simulink model "power_10MW5_diode"  (R2023b)
settings: Solver=FixedStepDiscrete  StartTime=0.0  StopTime=2.6  RelTol=1e-3
InitFcn:
  | power_sysinit
StopFcn:
  | ans = [pl_T1(end),max(tem_T1),pl_T2(end),max(tem_T2),pl_D1(end),max(tem_D1),...
  |     pl_D2(end),max(tem_D2),pl_D5(end),max(tem_D5),i_45(end),i_15(end),pl_D7(end),max(tem_D7)]
values from neighbouring files (symbols this model uses):
  C_absorption = 34e-6    (= 3.4e-05)    [power_sysinit.m]
  f = 40    [power_sysinit.m]
  f_switch = 900    [power_sysinit.m]
  IN = 0.3    [power_sysinit.m]
  L_absorption = 4e-6    (= 4e-06)    [power_sysinit.m]
  m = 1/75*f    (= 0.533333333333)    [power_sysinit.m]
  PM = 0    [power_sysinit.m]
  R_absorption = 0.45    [power_sysinit.m]
  TC = 1/f_switch    (= 0.00111111111111)    [power_sysinit.m]
  temp_init = 40    [power_sysinit.m]
  Ts1 = 1e-6    (= 1e-06)    [power_sysinit.m]
  Ts2 = 500E-6    (= 0.0005)    [power_sysinit.m]
  Udc = 2500    [power_sysinit.m]
undefined symbols (not defined in the file or in its folder): DIODE_204520, DIODE_344520, DIODE_364520, DIODE_364521, DIODE_D1031SH, DIODE_D1331SH, IGCT_364520_36, IGCT_364521_36, IGCT_654522_6, magnitude, Rth_h, Rth_h_tau
libraries: spsMeanLib x138, simulink x32, spsSeriesRLCBranchLib x30, spsRMSLib x24, spsCurrentMeasurementLib x21, dspstat3 x13, spsDiodeLib x12, spsVoltageMeasurementLib x12, spsOnDelayLib x6, powerlib_extras x5, spsDCVoltageSourceLib x4, spsIGBTDiodeLib x4
(part 1 of 6)
settings Model: SimulationMode=accelerator  Creator=tk  LastModifiedBy=Jhchen
settings SolverCC: AlgebraicLoopSolver=TrustRegion
settings DataIOCC: ReturnWorkspaceOutputs=off
settings OptimizationCC: EfficientMapNaN2IntZero=off
settings DebuggingCC: UnconnectedInputMsg=warning  UnconnectedOutputMsg=warning  UnconnectedLineMsg=warning  ArithmeticOperatorsInVariantConditions=warning
settings HardwareCC: TargetBitPerPointer=64  TargetBitPerSizeT=64  TargetBitPerPtrDiffT=64  TargetLongLongMode=on  TargetIntDivRoundTo=Zero  TargetEndianess=LittleEndian  TargetWordSize=64  TargetHWDeviceType=MATLAB Host  ProdEqTarget=off
settings ModelReferenceCC: EnableRefExpFcnMdlSchedulingChecks=on
settings SFSimCC: CustomCodeUndefinedFunction=UseInterfaceOnly
settings RTWCC: DLArmComputeVersion=19.05
settings CodeAppCC: MaxIdLength=128
settings GRTTargetCC: TargetLangStandard=C89/C90 (ANSI)  CombineOutputUpdateFcns=off  GRTInterface=on

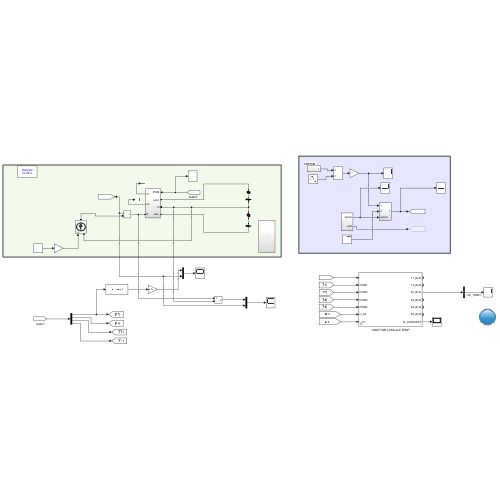
[thumbnail: Simulink's stored preview of the top-level diagram]
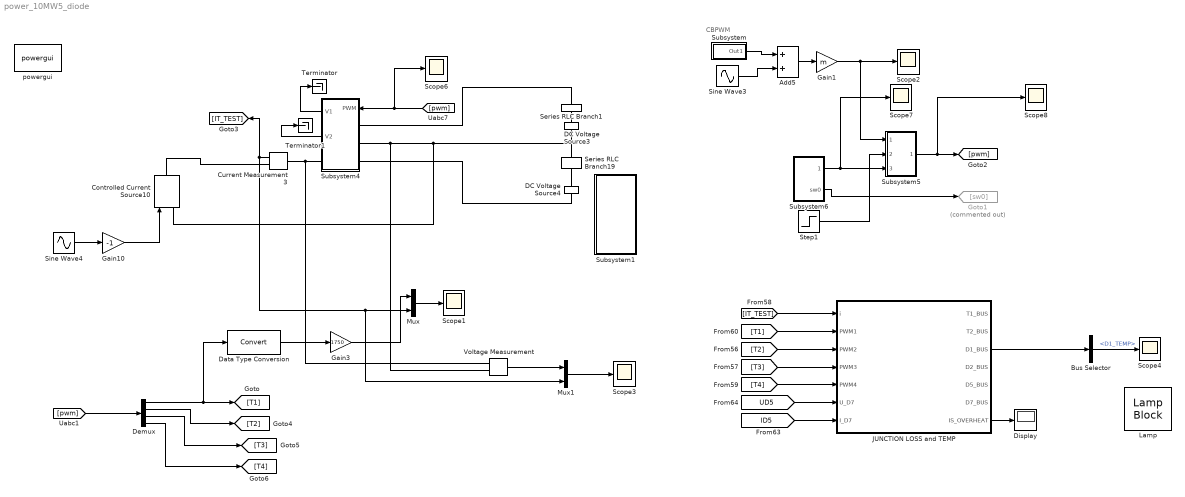
== system power_10MW5_diode ==
  note: CBPWM
  Add5 : Sum
  Bus Selector : BusSelector  OutputSignals=D1_TEMP
  Controlled Current Source10 : spsControlledCurrentSourceLib/Controlled Current Source  Initialize=on  Source_Type=DC  Amplitude=0  Phase=0  Frequency=0  Measurements=None
  Current Measurement3 : spsCurrentMeasurementLib/Current Measurement  PhasorSimulation=off  OutputType=Complex  PSBequivalent=0
  DC Voltage Source3 : spsDCVoltageSourceLib/DC Voltage Source  Amplitude=2500  Measurements=None
  DC Voltage Source4 : spsDCVoltageSourceLib/DC Voltage Source  Amplitude=2500  Measurements=None
  Data Type Conversion : DataTypeConversion  SaturateOnIntegerOverflow=off  RndMeth=Floor
  Demux : Demux
  Display : Display
  Gain1 : Gain  Gain=m
  Gain10 : Gain  Gain=-1
  Gain3 : Gain  Gain=1750
  Goto1 : Goto  Commented=on  GotoTag=sw0
  JUNCTION LOSS and TEMP : Subsystem  mask{DIODE_TYPE=34L4520, IGCT_TYPE=65l4522}
      mask prompts: DIODE_TYPE "DIODE"; IGCT_TYPE "IGCT"
      mask TypeOptions IGCT_TYPE: 65l4522 | 36L4520 | 36L4521
      mask DialogControl DescGroupVar Prompt: JUNCTION LOSS and TEMP
      mask DialogControl DescTextVar Prompt: 功率器件损耗与结温估算模块。通过下拉菜单选择相应IGCT与二极管
      mask DialogControl ParameterGroupVar Prompt: 参数
      mask DialogControl Container4 Prompt: IGCT型号，其中36L4520与36L4521为二极管和IGCT共用
  Lamp : LampBlock  LabelPosition=Hide
  Mux : Mux  Inputs=2
  Mux1 : Mux  Inputs=2
  Scope{1..4,6..8} (7 alike) : Scope
  Series RLC Branch1 : spsSeriesRLCBranchLib/Series RLC Branch  LConnTagsString=__new0  RConnTagsString=__new0  BranchType=R  Resistance=1E-6  Inductance=1e-3  SetiL0=off  InitialCurrent=0  Capacitance=1e-6  Setx0=off  InitialVoltage=0  Measurements=None
  Series RLC Branch19 : spsSeriesRLCBranchLib/Series RLC Branch  LConnTagsString=__new0  RConnTagsString=__new0  BranchType=R  Resistance=1E-6  Inductance=1e-3  SetiL0=off  InitialCurrent=0  Capacitance=1e-6  Setx0=off  InitialVoltage=0  Measurements=None
  Sine Wave3 : Sin  Frequency=2*f*pi  SampleTime=Ts2
  Sine Wave4 : Sin  Amplitude=IN*1750*1.4142  Frequency=2*f*pi  Phase=pi*(-0.05*f/50)  SampleTime=Ts1
  Step1 : Step  Time=0.00001  SampleTime=0
  Subsystem : Subsystem
  Subsystem1 : Subsystem
  Subsystem4 : Subsystem
  Subsystem5 : Subsystem
  Subsystem6 : Subsystem
  Terminator : Terminator
  Terminator1 : Terminator
  Voltage Measurement : spsVoltageMeasurementLib/Voltage Measurement  PhasorSimulation=off  OutputType=Complex  PSBequivalent=0
  powergui : sps_lib/powergui  Priority=1  SimulationMode=Discrete  SampleTime=1e-6  frequency=60  Iterations=50  frequencyindice=0  Pbase=100e6  ErrMax=1e-4  UnitsV=kV  UnitsW=MW  buscounter=0  FunctionMessages=off  echomessages=off  EnableUseOfTLC=off  CurrentSourceSwitches=off  DisableSnubberDevices=off  DisableRonSwitches=off  DisableVfSwitches=off  DisplayEquations=off  AutomaticDiscreteSolvers=off  SolverType=Tustin/Backward Euler (TBE)  Interpol=off  ExternalGateDelay=off  methode=off  Ts=100  x0status=blocks  SPID=off  SwTol=0  HookPort=off  NonlinearTolerance=1e-4  nMaxIteration=100  ContinueOnMaxIteration=off  RestoreLinks=warning  ResistiveCurrentMeasurement=off  Frange=[0:2:500]  Ylog=off  Xlog=on  ShowGrid=off  save=off  variable=ZData  structure=Iabc  ZoomFFT=off  StartTime=5.3  cycles=1  DisplayStyle=2  fundamental=47.875  FreqAxis=off  MaxFrequency=2000  frequencyindicesteady=1  RmsSteady=1  display=off
  wires:
  [pwm] -> Scope6/1, Subsystem4/1(PWM)
  Subsystem6/2(sw0) -> Goto1/1
  Step1/1 -> Subsystem5/2(In2)
  Subsystem6/1(carrier) -> Scope7/1, Subsystem5/3(carrier)
  Subsystem5/1(Out1) -> [pwm], Scope8/1
  Sine Wave4/1 -> Gain10/1
  Current Measurement3/1 -> [IT_TEST], Mux1/2, Mux/2
  Demux/4 -> [T4]
  [pwm] -> Demux/1
  Demux/1 -> Data Type Conversion/1, [T1]
  Demux/3 -> [T3]
  Demux/2 -> [T2]
  Mux/1 -> Scope1/1
  Sine Wave3/1 -> Add5/2
  Add5/1 -> Gain1/1
  Gain1/1 -> Subsystem5/1(In1), Scope2/1
  Data Type Conversion/1 -> Gain3/1
  Gain3/1 -> Mux/1
  Gain10/1 -> Controlled Current Source10/1
  Mux1/1 -> Scope3/1
  Voltage Measurement/1 -> Mux1/1
  Subsystem/1(Out1) -> Add5/1
  Subsystem4/1(V1) -> Terminator/1
  Subsystem4/2(V2) -> Terminator1/1
  [T4] -> JUNCTION LOSS and TEMP/5(PWM4)
  [T3] -> JUNCTION LOSS and TEMP/4(PWM3)
  [UD5] -> JUNCTION LOSS and TEMP/6(U_D7)
  [T2] -> JUNCTION LOSS and TEMP/3(PWM2)
  [ID5] -> JUNCTION LOSS and TEMP/7(I_D7)
  [T1] -> JUNCTION LOSS and TEMP/2(PWM1)
  [IT_TEST] -> JUNCTION LOSS and TEMP/1(i)
  JUNCTION LOSS and TEMP/7(IS_OVERHEAT) -> Display/1
  JUNCTION LOSS and TEMP/3(D1_BUS) -> Bus Selector/1
  Bus Selector/1 -> Scope4/1  "<D1_TEMP>"
  connections:
  Controlled Current Source10/LConn1 -- Series RLC Branch19/LConn1 -- DC Voltage Source3/LConn1 -- Voltage Measurement/LConn2 -- Subsystem4/LConn2
  Series RLC Branch1/LConn1 -- Subsystem4/LConn1
  Current Measurement3/LConn1 -- Voltage Measurement/LConn1 -- Subsystem4/RConn1
  DC Voltage Source4/LConn1 -- Subsystem4/LConn3
  DC Voltage Source4/RConn1 -- Series RLC Branch19/RConn1
  DC Voltage Source3/RConn1 -- Series RLC Branch1/RConn1
  Controlled Current Source10/RConn1 -- Current Measurement3/RConn1

== system power_10MW5_diode/JUNCTION LOSS and TEMP ==
  i : Inport
  PWM1 : Inport  Port=2
  PWM2 : Inport  Port=3
  PWM3 : Inport  Port=4
  PWM4 : Inport  Port=5
  U_D7 : Inport  Port=6
  I_D7 : Inport  Port=7
  Constant16 : Constant  Value=0
  DIODE : Subsystem  Variant=on
  Data Type Conversion4 : DataTypeConversion  OutDataTypeStr=boolean  SaturateOnIntegerOverflow=off  RndMeth=Floor
  IGCT : Subsystem  Variant=on  VariantControl=Variant Subsystem
  Logical Operator : Logic  Operator=OR  AllPortsSameDT=off  OutDataTypeStr=boolean
  S-R Flip-Flop : simulink_extras/Flip Flops/S-R Flip-Flop  initial_condition=0
  Terminator2 : Terminator
  To Workspace : ToWorkspace  VariableName=tem_T1  SampleTime=-1
  To Workspace1 : ToWorkspace  VariableName=pl_T1  SampleTime=-1
  To Workspace10 : ToWorkspace  VariableName=tem_D7  SampleTime=-1
  To Workspace11 : ToWorkspace  VariableName=pl_D7  SampleTime=-1
  To Workspace2 : ToWorkspace  VariableName=tem_D1  SampleTime=-1
  To Workspace3 : ToWorkspace  VariableName=pl_D1  SampleTime=-1
  To Workspace4 : ToWorkspace  VariableName=tem_T2  SampleTime=-1
  To Workspace5 : ToWorkspace  VariableName=pl_T2  SampleTime=-1
  To Workspace6 : ToWorkspace  VariableName=tem_D2  SampleTime=-1
  To Workspace7 : ToWorkspace  VariableName=pl_D2  SampleTime=-1
  To Workspace8 : ToWorkspace  VariableName=tem_D5  SampleTime=-1
  To Workspace9 : ToWorkspace  VariableName=pl_D5  SampleTime=-1
  T1_BUS : Outport
  T2_BUS : Outport  Port=2
  D1_BUS : Outport  Port=3
  D2_BUS : Outport  Port=4
  D5_BUS : Outport  Port=5
  D7_BUS : Outport  Port=6
  IS_OVERHEAT : Outport  Port=7
  wires:
  PWM1/1 -> DIODE/2(PWM1), IGCT/2(pwm1)
  DIODE/6(<D2_TEMP>) -> To Workspace6/1
  IGCT/3(<T1_TEMP>) -> To Workspace/1
  IGCT/7(TEMLIM_BOOL) -> Logical Operator/1
  DIODE/2(D2_BUS) -> D2_BUS/1
  IGCT/5(<T1_LOSS_MEAN>) -> To Workspace1/1
  S-R Flip-Flop/1 -> IS_OVERHEAT/1  "IS_OVERHEAT"
  DIODE/4(D7_BUS) -> D7_BUS/1
  DIODE/9(<D1_LOSS_MEAN>) -> To Workspace3/1
  i/1 -> DIODE/1(i), IGCT/1(i)
  IGCT/4(<T2_TEMP>) -> To Workspace4/1
  DIODE/8(<D7_TEMP>) -> To Workspace10/1
  PWM2/1 -> DIODE/3(PWM2), IGCT/3(pwm2)
  DIODE/5(<D1_TEMP>) -> To Workspace2/1
  IGCT/6(<T2_LOSS_MEAN>) -> To Workspace5/1
  S-R Flip-Flop/2 -> Terminator2/1
  DIODE/10(<D2_LOSS_MEAN>) -> To Workspace7/1
  DIODE/11(<D5_LOSS_MEAN>) -> To Workspace9/1
  U_D7/1 -> DIODE/6(U_D7)
  DIODE/3(D5_BUS) -> D5_BUS/1
  DIODE/13(TEMLIM_BOOL_D) -> Logical Operator/2
  IGCT/1(T1_BUS) -> T1_BUS/1
  DIODE/12(<D7_LOSS_MEAN>) -> To Workspace11/1
  DIODE/7(<D5_TEMP>) -> To Workspace8/1
  Constant16/1 -> Data Type Conversion4/1
  Data Type Conversion4/1 -> S-R Flip-Flop/2
  Logical Operator/1 -> S-R Flip-Flop/1
  DIODE/1(D1_BUS) -> D1_BUS/1
  IGCT/2(T2_BUS) -> T2_BUS/1
  I_D7/1 -> DIODE/7(I_D7)
  PWM3/1 -> DIODE/4(PWM3)
  PWM4/1 -> DIODE/5(PWM4)

== system power_10MW5_diode/Subsystem ==
  Add4 : Sum
  Gain : Gain  Gain=-0.5
  MinMax : MinMax  Inputs=3
  MinMax1 : MinMax  Function=max  Inputs=3
  Sine Wave1 : Sin  Frequency=2*f*pi  SampleTime=Ts2
  Sine Wave2 : Sin  Frequency=2*f*pi  Phase=2/3*pi  SampleTime=Ts2
  Sine Wave5 : Sin  Frequency=2*f*pi  Phase=4/3*pi  SampleTime=Ts2
  Out1 : Outport
  wires:
  Sine Wave1/1 -> MinMax1/1, MinMax/1
  MinMax/1 -> Add4/1
  Sine Wave5/1 -> MinMax1/3, MinMax/3
  Sine Wave2/1 -> MinMax1/2, MinMax/2
  MinMax1/1 -> Add4/2
  Add4/1 -> Gain/1
  Gain/1 -> Out1/1

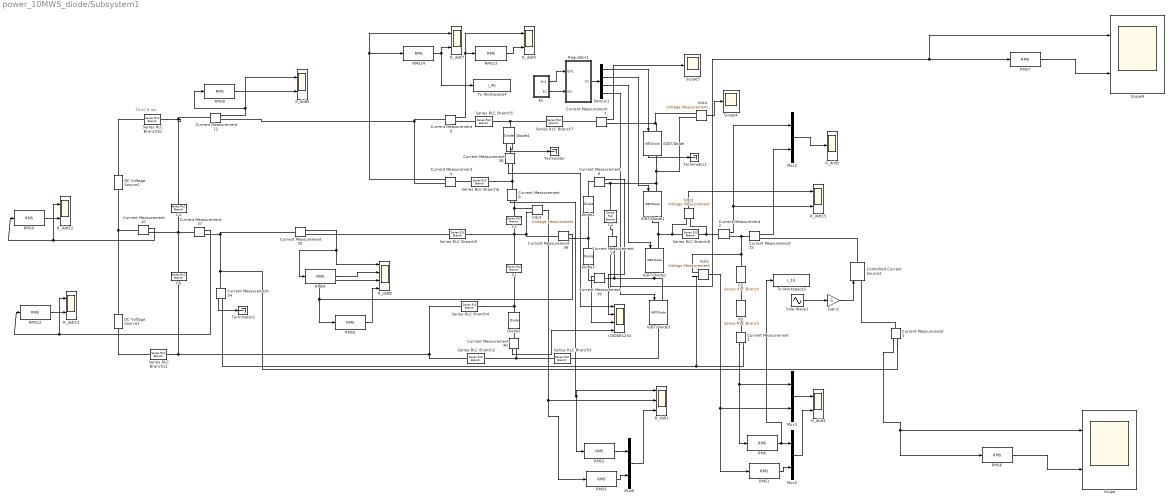
== system power_10MW5_diode/Subsystem1 ==
  note: TA=0.8 ms
  C1 : spsSeriesRLCBranchLib/Series RLC Branch  LConnTagsString=__new0  RConnTagsString=__new0  BranchType=C  Resistance=1.0  Inductance=1.0  SetiL0=off  InitialCurrent=0  Capacitance=C_absorption  Setx0=on  InitialVoltage=2400  Measurements=None
  C2 : spsSeriesRLCBranchLib/Series RLC Branch  LConnTagsString=__new0  RConnTagsString=__new0  BranchType=R  Resistance=12600  Inductance=1.0  SetiL0=off  InitialCurrent=0  Capacitance=1e-5  Setx0=on  InitialVoltage=2400  Measurements=None
  C3 : spsSeriesRLCBranchLib/Series RLC Branch  LConnTagsString=__new0  RConnTagsString=__new0  BranchType=C  Resistance=1.0  Inductance=1.0  SetiL0=off  InitialCurrent=0  Capacitance=C_absorption  Setx0=on  InitialVoltage=2400  Measurements=None
  C4 : spsSeriesRLCBranchLib/Series RLC Branch  LConnTagsString=__new0  RConnTagsString=__new0  BranchType=C  Resistance=1.0  Inductance=1.0  SetiL0=off  InitialCurrent=0  Capacitance=8e-3  Setx0=on  InitialVoltage=2580  Measurements=None
  C5 : spsSeriesRLCBranchLib/Series RLC Branch  LConnTagsString=__new0  RConnTagsString=__new0  BranchType=C  Resistance=2.25  Inductance=1e-6  SetiL0=off  InitialCurrent=0  Capacitance=0.625e-6  Setx0=off  InitialVoltage=0  Measurements=None
  C6 : spsSeriesRLCBranchLib/Series RLC Branch  LConnTagsString=__new0  RConnTagsString=__new0  BranchType=C  Resistance=1.0  Inductance=1.0  SetiL0=off  InitialCurrent=0  Capacitance=8e-3  Setx0=on  InitialVoltage=2580  Measurements=None
  Controlled Current Source1 : spsControlledCurrentSourceLib/Controlled Current Source  Initialize=on  Source_Type=DC  Amplitude=0  Phase=0  Frequency=0  Measurements=None
  Current Measurement{1..2,4..12,15,34..40} (19 alike) : spsCurrentMeasurementLib/Current Measurement  PhasorSimulation=off  OutputType=Complex  PSBequivalent=0
  DC Voltage Source1 : spsDCVoltageSourceLib/DC Voltage Source  Amplitude=2580  Measurements=None
  DC Voltage Source2 : spsDCVoltageSourceLib/DC Voltage Source  Amplitude=2580  Measurements=None
  Demux1 : Demux
  Diode2 : spsDiodeLib/Diode  Ron=0.001  Lon=0  Vf=0.8  IC=0  UseSnubber=off  Rs=5000  Cs=250e-9  Measurements=off
  Diode3 : spsDiodeLib/Diode  Ron=0.001  Lon=0  Vf=0.8  IC=0  UseSnubber=off  Rs=5000  Cs=250e-9  Measurements=off
  Diode4 : spsDiodeLib/Diode  Ron=0.001  Lon=0  Vf=0.8  IC=0  UseSnubber=off  Rs=500  Cs=250e-9  Measurements=on
  Diode5 : spsDiodeLib/Diode  Ron=0.001  Lon=0  Vf=0.8  IC=0  UseSnubber=off  Rs=500  Cs=250e-9  Measurements=off
  En : Subsystem
  Gain2 : Gain  Gain=-1
  I DIODE1234 : Scope  NumInputPorts=4
  IGBT/Diode : spsIGBTDiodeLib/IGBT//Diode  Ron=1e-3  Rs=500  Cs=1e-7  Measurements=on
  IGBT/Diode1 : spsIGBTDiodeLib/IGBT//Diode  Ron=1e-3  Rs=500  Cs=1e-7  Measurements=off
  IGBT/Diode2 : spsIGBTDiodeLib/IGBT//Diode  Ron=1e-3  Rs=500  Cs=1e-7  Measurements=off
  IGBT/Diode3 : spsIGBTDiodeLib/IGBT//Diode  Ron=1e-3  Rs=500  Cs=1e-7  Measurements=off
  Mux{2..3,5..6} (4 alike) : Mux  Inputs=2
  R1 : spsSeriesRLCBranchLib/Series RLC Branch  LConnTagsString=__new0  RConnTagsString=__new0  BranchType=R  Resistance=1.5  Inductance=1e-6  SetiL0=off  InitialCurrent=0  Capacitance=7e-7  Setx0=off  InitialVoltage=0  Measurements=None
  RMS : dspstat3/RMS  run=on  directionMode=Specified dimension  dimension=1  InputProcessing=Columns as channels (frame based)  reset_popup=None
  RMS1 : dspstat3/RMS  run=on  directionMode=Entire input  dimension=1  InputProcessing=Columns as channels (frame based)  reset_popup=None
  RMS{2..5,8..9,12..14} (9 alike) : dspstat3/RMS  run=on  directionMode=Each column  dimension=1  InputProcessing=Columns as channels (frame based)  reset_popup=None
  RMS6 : dspstat3/RMS  run=on  directionMode=Specified dimension  dimension=1  InputProcessing=Columns as channels (frame based)  reset_popup=None
  RMS7 : dspstat3/RMS  run=on  directionMode=Specified dimension  dimension=1  InputProcessing=Columns as channels (frame based)  reset_popup=None
  R_didt1 : Scope  NumInputPorts=3
  R_didt{3..5,7,12..13,15} (7 alike) : Scope  NumInputPorts=2
  R_didt2 : Scope
  R_didt8 : Scope  NumInputPorts=4
  Regulator1 : Subsystem  mask{TA=1/f_switch, Ts=Ts1, fn=50, KiP=3, LimI=0.3, Ur=1}
      mask prompts: TA "Control Sample Time [s]"; Ts "Power side sample time [s]"; fn "rated frequence [Hz]"; KiP "I adiuster P Coe."; LimI "I adjuster Output Lim."; Ur "Voltage ref. [pu]"
  Scope : Scope  NumInputPorts=2
  Scope4 : Scope
  Scope5 : Scope
  Scope9 : Scope  NumInputPorts=2
  Series RLC Branch10 : spsSeriesRLCBranchLib/Series RLC Branch  LConnTagsString=__new0  RConnTagsString=__new0  BranchType=RL  Resistance=1e-6  Inductance=0.5e-6  SetiL0=off  InitialCurrent=0  Capacitance=1e-6  Setx0=off  InitialVoltage=0  Measurements=None
  Series RLC Branch11 : spsSeriesRLCBranchLib/Series RLC Branch  LConnTagsString=__new0  RConnTagsString=__new0  BranchType=RL  Resistance=1e-6  Inductance=0.5e-6  SetiL0=off  InitialCurrent=0  Capacitance=1e-6  Setx0=off  InitialVoltage=0  Measurements=None
  Series RLC Branch2 : spsSeriesRLCBranchLib/Series RLC Branch  LConnTagsString=__new0  RConnTagsString=__new0  BranchType=L  Resistance=1  Inductance=L_absorption  SetiL0=off  InitialCurrent=0  Capacitance=1e-6  Setx0=off  InitialVoltage=0  Measurements=None
  Series RLC Branch3 : spsSeriesRLCBranchLib/Series RLC Branch  LConnTagsString=__new0  RConnTagsString=__new0  BranchType=L  Resistance=1  Inductance=0.1e-6  SetiL0=off  InitialCurrent=0  Capacitance=1e-6  Setx0=off  InitialVoltage=0  Measurements=None
  Series RLC Branch4 : spsSeriesRLCBranchLib/Series RLC Branch  LConnTagsString=__new0  RConnTagsString=__new0  BranchType=R  Resistance=R_absorption  Inductance=7e-6  SetiL0=off  InitialCurrent=0  Capacitance=1e-6  Setx0=off  InitialVoltage=0  Measurements=Branch voltage and current
  Series RLC Branch5 : spsSeriesRLCBranchLib/Series RLC Branch  LConnTagsString=__new0  RConnTagsString=__new0  BranchType=L  Resistance=1  Inductance=L_absorption  SetiL0=off  InitialCurrent=0  Capacitance=1e-6  Setx0=off  InitialVoltage=0  Measurements=None
  Series RLC Branch6 : spsSeriesRLCBranchLib/Series RLC Branch  LConnTagsString=__new0  RConnTagsString=__new0  BranchType=R  Resistance=R_absorption  Inductance=7e-6  SetiL0=off  InitialCurrent=0  Capacitance=1e-6  Setx0=off  InitialVoltage=0  Measurements=None
  Series RLC Branch7 : spsSeriesRLCBranchLib/Series RLC Branch  LConnTagsString=__new0  RConnTagsString=__new0  BranchType=L  Resistance=1  Inductance=0.1e-6  SetiL0=off  InitialCurrent=0  Capacitance=1e-6  Setx0=off  InitialVoltage=0  Measurements=None
  Series RLC Branch8 : spsSeriesRLCBranchLib/Series RLC Branch  LConnTagsString=__new0  RConnTagsString=__new0  BranchType=L  Resistance=1  Inductance=L_absorption  SetiL0=off  InitialCurrent=0  Capacitance=1e-6  Setx0=off  InitialVoltage=0  Measurements=Branch voltage
  Series RLC Branch9 : spsSeriesRLCBranchLib/Series RLC Branch  LConnTagsString=__new0  RConnTagsString=__new0  BranchType=L  Resistance=1  Inductance=0.5e-6  SetiL0=off  InitialCurrent=0  Capacitance=1e-6  Setx0=off  InitialVoltage=0  Measurements=None
  Sine Wave1 : Sin  Amplitude=1*IN*1750*1.4142  Frequency=2*f*pi  Phase=-pi*(0.05*50/50)  SampleTime=Ts1
  Terminator : Terminator
  Terminator1 : Terminator
  Terminator2 : Terminator
  To Workspace4 : ToWorkspace  VariableName=i_45  SampleTime=-1
  To Workspace5 : ToWorkspace  VariableName=i_15  SampleTime=-1
  Vdc{1..4} (4 alike) : spsVoltageMeasurementLib/Voltage Measurement  Tag=PoWeRsYsTeMmEaSuReMeNt  PhasorSimulation=off  OutputType=Magnitude  PSBequivalent=0
  wires:
  RMS8/1 -> R_didt4/2
  Demux1/2 -> IGBT/Diode1/1
  Mux2/1 -> R_didt2/1
  Current Measurement36/1 -> R_didt8/3, RMS5/1
  Mux3/1 -> R_didt3/1
  Current Measurement15/1 -> Mux2/2
  Current Measurement5/1 -> RMS/1, Mux3/1
  Current Measurement38/1 -> I DIODE1234/1
  Demux1/4 -> IGBT/Diode3/1
  Current Measurement9/1 -> RMS13/1, R_didt5/1
  Current Measurement35/1 -> RMS4/1, R_didt8/1
  Current Measurement34/1 -> Terminator2/1
  RMS5/1 -> R_didt8/4
  Current Measurement40/1 -> I DIODE1234/4
  Mux6/1 -> R_didt1/3
  Current Measurement39/1 -> I DIODE1234/3
  Vdc3/1 -> RMS3/1, R_didt1/2
  En/1(En1) -> Regulator1/1(EN1)
  RMS7/1 -> Scope9/2
  Demux1/1 -> IGBT/Diode/1
  Demux1/3 -> IGBT/Diode2/1
  Current Measurement2/1 -> R_didt15/2, Mux2/1
  Current Measurement10/1 -> RMS9/1, R_didt12/1
  Current Measurement12/1 -> R_didt4/1, RMS8/1
  Vdc1/1 -> RMS1/1, Mux3/2
  Sine Wave1/1 -> Gain2/1
  Current Measurement6/1 -> I DIODE1234/2
  RMS14/1 -> R_didt7/2, To Workspace4/1
  Current Measurement11/1 -> Scope9/1, RMS7/1
  RMS9/1 -> R_didt12/2
  Gain2/1 -> Controlled Current Source1/1
  RMS12/1 -> R_didt13/2
  Current Measurement4/1 -> RMS14/1, R_didt7/1
  Vdc4/1 -> Scope4/1
  RMS6/1 -> Scope/2
  Mux5/1 -> R_didt3/2
  Current Measurement7/1 -> Scope5/1
  Vdc2/1 -> R_didt15/1
  RMS3/1 -> Mux6/2
  Current Measurement1/1 -> RMS6/1, Scope/1
  RMS4/1 -> R_didt8/2
  RMS1/1 -> Mux5/2
  Current Measurement8/1 -> RMS2/1, R_didt1/1
  RMS2/1 -> Mux6/1
  En/2(En) -> Regulator1/2(EN)
  RMS/1 -> To Workspace5/1, Mux5/1
  Current Measurement37/1 -> RMS12/1, R_didt13/1
  RMS13/1 -> R_didt5/2
  Regulator1/1(P2) -> Demux1/1
  Diode4/1 -> Terminator/1
  IGBT/Diode/1 -> Terminator1/1
  connections:
  Controlled Current Source1/RConn1 -- Current Measurement15/RConn1
  Vdc2/LConn2 -- Current Measurement2/LConn1 -- Series RLC Branch8/LConn1
  Current Measurement15/LConn1 -- C5/LConn1 -- Vdc1/LConn1 -- Current Measurement2/RConn1
  Current Measurement36/LConn1 -- C1/LConn1 -- C3/RConn1 -- Series RLC Branch9/RConn1 -- Vdc3/LConn2
  Current Measurement1/LConn1 -- Controlled Current Source1/LConn1
  Series RLC Branch4/RConn1 -- C1/RConn1 -- Diode5/LConn1
  Series RLC Branch2/LConn1 -- Series RLC Branch4/LConn1 -- Series RLC Branch11/RConn1 -- C6/RConn1
  Current Measurement10/RConn1 -- C4/RConn1 -- Current Measurement37/LConn1 -- C6/LConn1
  Current Measurement38/RConn1 -- Series RLC Branch6/RConn1 -- Current Measurement8/LConn1
  Series RLC Branch10/LConn1 -- DC Voltage Source2/RConn1
  IGBT/Diode3/RConn1 -- Series RLC Branch3/RConn1
  Current Measurement34/LConn1 -- Current Measurement37/RConn1 -- Current Measurement35/LConn1 -- Current Measurement1/RConn1
  DC Voltage Source1/LConn1 -- Series RLC Branch11/LConn1
  Current Measurement7/LConn1 -- Series RLC Branch7/RConn1
  Current Measurement11/LConn1 -- C2/RConn1
  DC Voltage Source2/LConn1 -- DC Voltage Source1/RConn1 -- Current Measurement10/LConn1
  Current Measurement40/LConn1 -- Diode5/RConn1
  Current Measurement6/RConn1 -- IGBT/Diode/RConn1 -- Vdc4/LConn2 -- IGBT/Diode1/LConn1 -- C2/LConn1
  Diode3/RConn1 -- Diode2/LConn1 -- Current Measurement36/RConn1
  Current Measurement4/RConn1 -- Current Measurement12/RConn1 -- Current Measurement9/LConn1
  Current Measurement38/LConn1 -- Diode4/RConn1
  Series RLC Branch9/LConn1 -- Current Measurement35/RConn1
  Diode4/LConn1 -- Series RLC Branch5/RConn1 -- Series RLC Branch7/LConn1
  C4/LConn1 -- Series RLC Branch10/RConn1 -- Current Measurement12/LConn1
  Current Measurement39/RConn1 -- Diode3/LConn1
  IGBT/Diode/LConn1 -- Current Measurement7/RConn1 -- Vdc4/LConn1
  Current Measurement34/RConn1 -- Current Measurement5/RConn1 -- Vdc1/LConn2
  Vdc3/LConn1 -- Current Measurement8/RConn1 -- C3/LConn1
  Current Measurement5/LConn1 -- R1/LConn1
  R1/RConn1 -- C5/RConn1
  Current Measurement6/LConn1 -- Diode2/RConn1
  Current Measurement9/RConn1 -- Series RLC Branch5/LConn1
  Current Measurement4/LConn1 -- Series RLC Branch6/LConn1
  Series RLC Branch3/LConn1 -- Series RLC Branch2/RConn1 -- Current Measurement40/RConn1
  IGBT/Diode2/LConn1 -- Series RLC Branch8/RConn1 -- Vdc2/LConn1 -- IGBT/Diode1/RConn1
  Current Measurement39/LConn1 -- IGBT/Diode3/LConn1 -- IGBT/Diode2/RConn1 -- Current Measurement11/RConn1

== system power_10MW5_diode/Subsystem4 ==
  PWM : Inport
  Subsystem2 : Subsystem
  udc+ : PMIOPort  Side=Left
  N : PMIOPort  Port=2  Side=Left
  udc- : PMIOPort  Port=3  Side=Left
  B : PMIOPort  Port=4  Side=Right
  V1 : Outport  VectorParamsAs1DForOutWhenUnconnected=off
  V2 : Outport  Port=2  VectorParamsAs1DForOutWhenUnconnected=off
  wires:
  Subsystem2/1(V1) -> V1/1
  Subsystem2/2(V2) -> V2/1
  PWM/1 -> Subsystem2/1(PWM)
  connections:
  Subsystem2/RConn1 -- B/RConn1
  Subsystem2/LConn2 -- N/RConn1
  Subsystem2/LConn3 -- udc-/RConn1
  Subsystem2/LConn1 -- udc+/RConn1

== system power_10MW5_diode/Subsystem5 ==
  In1 : Inport
  In2 : Inport  Port=2
  carrier : Inport  Port=3
  Bitwise Operator : simulink/Logic and Bit Operations/Bitwise Operator  logicop=NOT  UseBitMask=off  BitMask=bin2dec('11011001')  BitMaskRealWorld=Stored Integer
  Bitwise Operator1 : simulink/Logic and Bit Operations/Bitwise Operator  logicop=NOT  UseBitMask=off  BitMask=bin2dec('11011001')  BitMaskRealWorld=Stored Integer
  Demux7 : Demux  Outputs=2
  Mux1 : Mux
  On Delay{,1..3} (4 alike) : spsOnDelayLib/On Delay  DelayType=On delay  delay=Td  ic=0  Ts=0
  Relational Operator : RelationalOperator  Operator=<=  OutDataTypeStr=boolean  InputSameDT=off
  Relational Operator1 : RelationalOperator  OutDataTypeStr=boolean  InputSameDT=off
  Scope5 : Scope
  Subsystem : Subsystem
  Out1 : Outport  VectorParamsAs1DForOutWhenUnconnected=off
  wires:
  Relational Operator/1 -> On Delay1/1, Bitwise Operator1/1
  Bitwise Operator1/1 -> On Delay2/1
  Bitwise Operator/1 -> On Delay3/1
  On Delay3/1 -> Subsystem/3(In3)
  On Delay1/1 -> Subsystem/4(In4)
  Subsystem/2(Out2) -> Mux1/2
  Subsystem/1(Out1) -> Mux1/1
  Subsystem/3(Out3) -> Mux1/3
  Subsystem/4(Out4) -> Mux1/4
  Mux1/1 -> Out1/1
  In2/1 -> Subsystem/5(INL)
  On Delay2/1 -> Subsystem/2(In2)
  On Delay/1 -> Subsystem/1(In1)
  In1/1 -> Relational Operator/1, Relational Operator1/1
  Relational Operator1/1 -> Bitwise Operator/1, On Delay/1
  Demux7/1 -> Relational Operator1/2
  Demux7/2 -> Relational Operator/2
  carrier/1 -> Scope5/1, Demux7/1

== system power_10MW5_diode/Subsystem6 ==
  note: only switch at the time carrier1=0&carrier2=0
  Abs : Abs  SaturateOnIntegerOverflow=off
  Abs1 : Abs  SaturateOnIntegerOverflow=off
  Add : Sum
  Add5 : Sum
  Add6 : Sum
  Constant : Constant  Value=-1
  Constant1 : Constant  Value=0.002
  Constant2 : Constant  Value=PM  OutDataTypeStr=boolean
  Constant5 : Constant  Value=-0.5
  Constant6 : Constant  Value=-1
  Data Type Conversion : DataTypeConversion  SaturateOnIntegerOverflow=off  RndMeth=Floor
  Delay : Delay  DelayLength=1  InitialCondition=0
  Logical Operator : Logic  AllPortsSameDT=off  OutDataTypeStr=boolean
  Mux1 : Mux  Inputs=2
  Mux15 : Mux  Inputs=2
  Mux16 : Mux  Inputs=2
  Mux2 : Mux  Inputs=3
  Relational Operator1 : RelationalOperator  Operator=<  OutDataTypeStr=boolean  RndMeth=Simplest  InputSameDT=off
  Relational Operator2 : RelationalOperator  Operator=<  OutDataTypeStr=boolean  RndMeth=Simplest  InputSameDT=off
  Repeating Sequence : simulink/Sources/Repeating Sequence  rep_seq_t=[0 TC/2 TC]  rep_seq_y=[0 1 0]
  Repeating Sequence1 : simulink/Sources/Repeating Sequence  rep_seq_t=[0 TC 2*TC]  rep_seq_y=[0 2 0]
  Repeating Sequence2 : simulink/Sources/Repeating Sequence  rep_seq_t=[0 TC 2*TC]  rep_seq_y=[0 2 0]
  Repeating Sequence3 : simulink/Sources/Repeating Sequence  rep_seq_t=[0 TC/2 TC]  rep_seq_y=[0 1 0]
  Scope{,1..3} (4 alike) : Scope
  Switch : Switch  Criteria=u2 > Threshold  SaturateOnIntegerOverflow=off  InputSameDT=off
  Switch1 : Switch  Criteria=u2 > Threshold  SaturateOnIntegerOverflow=off  InputSameDT=off
  carrier : Outport  VectorParamsAs1DForOutWhenUnconnected=off
  sw0 : Outport  Port=2  VectorParamsAs1DForOutWhenUnconnected=off
  wires:
  Add5/1 -> Mux16/1
  Constant2/1 -> Switch1/1, Mux1/2
  Repeating Sequence2/1 -> Add6/1
  Repeating Sequence1/1 -> Abs1/1, Mux2/2, Add5/1
  Mux16/1 -> Switch/3
  Repeating Sequence/1 -> Add/1
  Constant5/1 -> Add5/2
  Constant6/1 -> Add6/2
  Mux15/1 -> Switch/1
  Add/1 -> Mux15/2
  Constant/1 -> Add/2
  Add6/1 -> Mux16/2
  Switch/1 -> Scope3/1, carrier/1
  Abs/1 -> Relational Operator1/1
  Abs1/1 -> Relational Operator2/1
  Constant1/1 -> Relational Operator2/2, Relational Operator1/2
  Relational Operator1/1 -> Logical Operator/1
  Relational Operator2/1 -> Logical Operator/2
  Repeating Sequence3/1 -> Abs/1, Mux2/1, Mux15/1
  Mux2/1 -> Scope1/1
  Switch1/1 -> Data Type Conversion/1, Delay/1, Scope/1, Switch/2, sw0/1
  Data Type Conversion/1 -> Mux2/3
  Logical Operator/1 -> Switch1/2, Mux1/1
  Mux1/1 -> Scope2/1
  Delay/1 -> Switch1/3

== system power_10MW5_diode/JUNCTION LOSS and TEMP/DIODE ==
  i : Inport
  PWM1 : Inport  Port=2
  PWM2 : Inport  Port=3
  PWM3 : Inport  Port=4
  PWM4 : Inport  Port=5
  U_D7 : Inport  Port=6
  I_D7 : Inport  Port=7
  20L4520 : Subsystem  VariantControl=DIODE_TYPE==1
  34L4520 : Subsystem  VariantControl=DIODE_TYPE==2
  36L4520_D : Subsystem  VariantControl=DIODE_TYPE==5
  36L4521_D : Subsystem  VariantControl=DIODE_TYPE==6
  D1031SH : Subsystem  VariantControl=DIODE_TYPE==3
  D1331SH : Subsystem  VariantControl=DIODE_TYPE==4
  D1_BUS : Outport
  D2_BUS : Outport  Port=2
  D5_BUS : Outport  Port=3
  D7_BUS : Outport  Port=4
  <D1_TEMP> : Outport  Port=5
  <D2_TEMP> : Outport  Port=6
  <D5_TEMP> : Outport  Port=7
  <D7_TEMP> : Outport  Port=8
  <D1_LOSS_MEAN> : Outport  Port=9
  <D2_LOSS_MEAN> : Outport  Port=10
  <D5_LOSS_MEAN> : Outport  Port=11
  <D7_LOSS_MEAN> : Outport  Port=12
  TEMLIM_BOOL_D : Outport  Port=13

== system power_10MW5_diode/JUNCTION LOSS and TEMP/IGCT ==
  i : Inport
  pwm1 : Inport  Port=2
  pwm2 : Inport  Port=3
  36L4520 : Subsystem  VariantControl=IGCT_TYPE==2
  36L4521 : Subsystem  VariantControl=IGCT_TYPE==3
  65L4522 : Subsystem  VariantControl=IGCT_TYPE==1
  T1_BUS : Outport
  T2_BUS : Outport  Port=2
  <T1_TEMP> : Outport  Port=3
  <T2_TEMP> : Outport  Port=4
  <T1_LOSS_MEAN> : Outport  Port=5
  <T2_LOSS_MEAN> : Outport  Port=6
  TEMLIM_BOOL : Outport  Port=7

== system power_10MW5_diode/Subsystem1/En ==
  On/Off Delay3 : powerlib_extras/Control  Blocks/On//Off Delay  type_delay=On delay  delay=0.001  ic=0
  Step : Step  Time=0.01  SampleTime=0  ZeroCross=off
  En1 : Outport
  En : Outport  Port=2
  wires:
  Step/1 -> En/1, On/Off Delay3/1
  On/Off Delay3/1 -> En1/1

== system power_10MW5_diode/Subsystem1/Regulator1 ==
  EN1 : Inport
  EN : Inport  Port=2
  1st order delay5 : Subsystem
  Constant : Constant
  Constant1 : Constant  Value=0
  Data Type Conversion : DataTypeConversion  SaturateOnIntegerOverflow=off  RndMeth=Floor
  Fis : Subsystem
  PWM2 : Subsystem
  Switch : Switch  Threshold=0.5  ZeroCross=off  SaturateOnIntegerOverflow=off  InputSameDT=off
  Vabc_r1 : Subsystem
  P2 : Outport
  wires:
  EN1/1 -> Data Type Conversion/1
  Data Type Conversion/1 -> Switch/2
  Constant/1 -> Switch/1
  Constant1/1 -> Switch/3
  Switch/1 -> 1st order delay5/1(x)
  Fis/1(Fis1) -> Vabc_r1/1(Fis)
  EN/1 -> PWM2/2(EN2), Fis/1(En)
  1st order delay5/1(y) -> Vabc_r1/2(Ur)
  PWM2/1(P1) -> P2/1
  Vabc_r1/1(Va) -> PWM2/1(Uref)

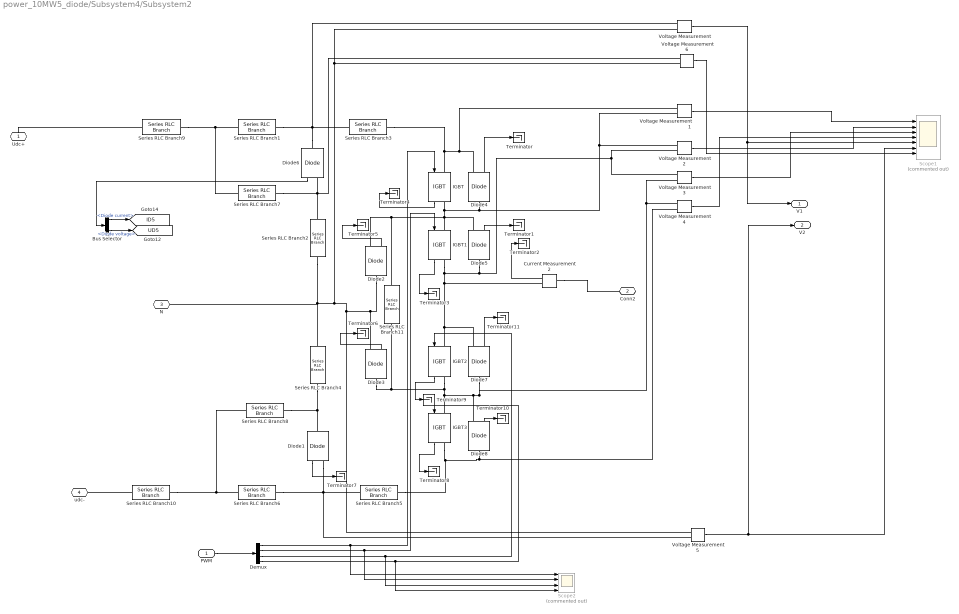
== system power_10MW5_diode/Subsystem4/Subsystem2 ==
  PWM : Inport
  Bus Selector : BusSelector  OutputSignals=Diode current,Diode voltage
  Current Measurement2 : spsCurrentMeasurementLib/Current Measurement  PhasorSimulation=off  OutputType=Complex  PSBequivalent=0
  Demux : Demux
  Diode{1..8} (8 alike) : spsDiodeLib/Diode  Ron=rF_DIODE  Lon=0  Vf=VT0_DIODE  IC=0  UseSnubber=off  Rs=500  Cs=250e-9  Measurements=on
  IGBT{,1..3} (4 alike) : spsIGBTLib/IGBT  Ron=rT_GCT  Lon=0  Vf=VT0_GCT  Tf=1e-6  Tt=2e-6  IC=0  Rs=1e5  Cs=inf  Measurements=on
  Scope1 : Scope  Commented=on  NumInputPorts=7
  Scope2 : Scope  Commented=on  NumInputPorts=4
  Series RLC Branch1 : spsSeriesRLCBranchLib/Series RLC Branch  LConnTagsString=__new0  RConnTagsString=__new0  BranchType=L  Resistance=1  Inductance=L_absorption  SetiL0=off  InitialCurrent=0  Capacitance=1e-6  Setx0=off  InitialVoltage=0  Measurements=None
  Series RLC Branch10 : spsSeriesRLCBranchLib/Series RLC Branch  LConnTagsString=__new0  RConnTagsString=__new0  BranchType=L  Resistance=1  Inductance=0.4e-8  SetiL0=off  InitialCurrent=0  Capacitance=1e-6  Setx0=off  InitialVoltage=0  Measurements=None
  Series RLC Branch11 : spsSeriesRLCBranchLib/Series RLC Branch  LConnTagsString=__new0  RConnTagsString=__new0  BranchType=R  Resistance=25E3  Inductance=20e-6  SetiL0=off  InitialCurrent=0  Capacitance=1e-6  Setx0=off  InitialVoltage=0  Measurements=None
  Series RLC Branch2 : spsSeriesRLCBranchLib/Series RLC Branch  LConnTagsString=__new0  RConnTagsString=__new0  BranchType=C  Resistance=1  Inductance=20e-6  SetiL0=off  InitialCurrent=0  Capacitance=C_absorption  Setx0=off  InitialVoltage=0  Measurements=None
  Series RLC Branch3 : spsSeriesRLCBranchLib/Series RLC Branch  LConnTagsString=__new0  RConnTagsString=__new0  BranchType=L  Resistance=1  Inductance=1E-10  SetiL0=off  InitialCurrent=0  Capacitance=1e-6  Setx0=off  InitialVoltage=0  Measurements=None
  Series RLC Branch4 : spsSeriesRLCBranchLib/Series RLC Branch  LConnTagsString=__new0  RConnTagsString=__new0  BranchType=C  Resistance=1  Inductance=20e-6  SetiL0=off  InitialCurrent=0  Capacitance=R_absorption  Setx0=off  InitialVoltage=0  Measurements=None
  Series RLC Branch5 : spsSeriesRLCBranchLib/Series RLC Branch  LConnTagsString=__new0  RConnTagsString=__new0  BranchType=L  Resistance=1  Inductance=1E-10  SetiL0=off  InitialCurrent=0  Capacitance=1e-6  Setx0=off  InitialVoltage=0  Measurements=None
  Series RLC Branch6 : spsSeriesRLCBranchLib/Series RLC Branch  LConnTagsString=__new0  RConnTagsString=__new0  BranchType=L  Resistance=1  Inductance=L_absorption  SetiL0=off  InitialCurrent=0  Capacitance=1e-6  Setx0=off  InitialVoltage=0  Measurements=None
  Series RLC Branch7 : spsSeriesRLCBranchLib/Series RLC Branch  LConnTagsString=__new0  RConnTagsString=__new0  BranchType=R  Resistance=R_absorption  Inductance=20e-6  SetiL0=off  InitialCurrent=0  Capacitance=1e-6  Setx0=off  InitialVoltage=0  Measurements=None
  Series RLC Branch8 : spsSeriesRLCBranchLib/Series RLC Branch  LConnTagsString=__new0  RConnTagsString=__new0  BranchType=R  Resistance=R_absorption  Inductance=20e-6  SetiL0=off  InitialCurrent=0  Capacitance=1e-6  Setx0=off  InitialVoltage=0  Measurements=None
  Series RLC Branch9 : spsSeriesRLCBranchLib/Series RLC Branch  LConnTagsString=__new0  RConnTagsString=__new0  BranchType=L  Resistance=1  Inductance=0.4e-8  SetiL0=off  InitialCurrent=0  Capacitance=1e-6  Setx0=off  InitialVoltage=0  Measurements=None
  Terminator{,1..11} (12 alike) : Terminator
  Voltage Measurement{,1..6} (7 alike) : spsVoltageMeasurementLib/Voltage Measurement  PhasorSimulation=off  OutputType=Complex  PSBequivalent=0
  Udc+ : PMIOPort  Side=Left
  Conn2 : PMIOPort  Port=2  Side=Right
  N : PMIOPort  Port=3  Side=Left
  udc- : PMIOPort  Port=4  Side=Left
  V1 : Outport  VectorParamsAs1DForOutWhenUnconnected=off
  V2 : Outport  Port=2  VectorParamsAs1DForOutWhenUnconnected=off
  tag scope: ID5=global, UD5=global
  wires:
  PWM/1 -> Demux/1
  Demux/1 -> Scope2/1, IGBT/1
  Demux/2 -> IGBT1/1, Scope2/2
  Demux/3 -> IGBT2/1, Scope2/3
  Demux/4 -> IGBT3/1, Scope2/4
  Voltage Measurement/1 -> V1/1, Scope1/5
  Voltage Measurement1/1 -> Scope1/1
  Voltage Measurement2/1 -> Scope1/2
  Voltage Measurement3/1 -> Scope1/3
  Voltage Measurement4/1 -> Scope1/4
  Voltage Measurement5/1 -> V2/1, Scope1/6
  Voltage Measurement6/1 -> Scope1/7
  Diode6/1 -> Bus Selector/1
  Bus Selector/2 -> [UD5]  "<Diode voltage>"
  Bus Selector/1 -> [ID5]  "<Diode current>"
  Diode4/1 -> Terminator/1
  Diode5/1 -> Terminator1/1
  Current Measurement2/1 -> Terminator2/1
  IGBT1/1 -> Terminator3/1
  IGBT/1 -> Terminator4/1
  Diode2/1 -> Terminator5/1
  Diode3/1 -> Terminator6/1
  Diode1/1 -> Terminator7/1
  IGBT3/1 -> Terminator8/1
  IGBT2/1 -> Terminator9/1
  Diode8/1 -> Terminator10/1
  Diode7/1 -> Terminator11/1
  connections:
  Voltage Measurement3/LConn1 -- Voltage Measurement2/LConn2 -- IGBT1/RConn1 -- Diode7/RConn1 -- IGBT2/LConn1 -- Current Measurement2/RConn1 -- Diode5/LConn1
  Diode6/LConn1 -- Voltage Measurement/LConn1 -- Series RLC Branch1/RConn1 -- Series RLC Branch3/LConn1
  Series RLC Branch5/LConn1 -- Diode1/RConn1 -- Voltage Measurement5/LConn2 -- Series RLC Branch6/RConn1
  Series RLC Branch6/LConn1 -- Series RLC Branch10/RConn1 -- Series RLC Branch8/LConn1
  Voltage Measurement5/LConn1 -- Diode2/LConn1 -- Diode3/RConn1 -- Voltage Measurement6/LConn2 -- Voltage Measurement/LConn2 -- Series RLC Branch4/LConn1 -- Series RLC Branch2/RConn1 -- N/RConn1
  Series RLC Branch1/LConn1 -- Series RLC Branch9/RConn1 -- Series RLC Branch7/LConn1
  Series RLC Branch11/RConn1 -- Diode3/LConn1 -- IGBT2/RConn1 -- IGBT3/LConn1 -- Voltage Measurement3/LConn2 -- Voltage Measurement4/LConn1 -- Diode7/LConn1 -- Diode8/RConn1
  Diode6/RConn1 -- Voltage Measurement6/LConn1 -- Series RLC Branch2/LConn1 -- Series RLC Branch7/RConn1
  Series RLC Branch11/LConn1 -- Diode2/RConn1 -- IGBT1/LConn1 -- Diode5/RConn1 -- Diode4/LConn1 -- Voltage Measurement2/LConn1 -- Voltage Measurement1/LConn2 -- IGBT/RConn1
  Series RLC Branch5/RConn1 -- IGBT3/RConn1 -- Diode8/LConn1 -- Voltage Measurement4/LConn2
  Series RLC Branch4/RConn1 -- Diode1/LConn1 -- Series RLC Branch8/RConn1
  Series RLC Branch3/RConn1 -- Diode4/RConn1 -- Voltage Measurement1/LConn1 -- IGBT/LConn1
  Series RLC Branch9/LConn1 -- Udc+/RConn1
  Series RLC Branch10/LConn1 -- udc-/RConn1
  Current Measurement2/LConn1 -- Conn2/RConn1

== system power_10MW5_diode/Subsystem5/Subsystem ==
  In1 : Inport
  In2 : Inport  Port=2
  In3 : Inport  Port=3
  In4 : Inport  Port=4
  INL : Inport  Port=5
  Logical Operator{,1..3} (4 alike) : Logic  AllPortsSameDT=off  OutDataTypeStr=boolean
  Off Delay : spsOnDelayLib/On Delay  DelayType=On delay  delay=5e-6  ic=1  Ts=0
  Off Delay1 : spsOnDelayLib/On Delay  DelayType=On delay  delay=5e-6  ic=1  Ts=0
  Out1 : Outport  VectorParamsAs1DForOutWhenUnconnected=off
  Out2 : Outport  Port=2  VectorParamsAs1DForOutWhenUnconnected=off
  Out3 : Outport  Port=3  VectorParamsAs1DForOutWhenUnconnected=off
  Out4 : Outport  Port=4  VectorParamsAs1DForOutWhenUnconnected=off
  wires:
  Off Delay/1 -> Logical Operator/2
  In2/1 -> Logical Operator/1
  Off Delay1/1 -> Logical Operator1/2
  In3/1 -> Logical Operator1/1
  INL/1 -> Logical Operator2/2, Off Delay/1, Off Delay1/1, Logical Operator3/2
  In1/1 -> Logical Operator2/1
  Logical Operator/1 -> Out2/1
  Logical Operator3/1 -> Out4/1
  Logical Operator2/1 -> Out1/1
  Logical Operator1/1 -> Out3/1
  In4/1 -> Logical Operator3/1

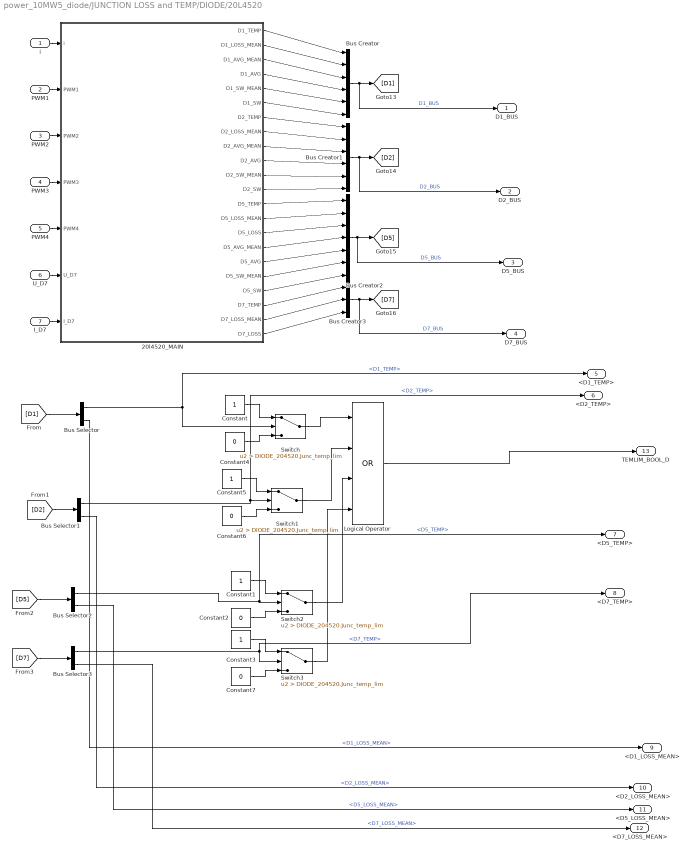
== system power_10MW5_diode/JUNCTION LOSS and TEMP/DIODE/20L4520 ==
  i : Inport
  PWM1 : Inport  Port=2
  PWM2 : Inport  Port=3
  PWM3 : Inport  Port=4
  PWM4 : Inport  Port=5
  U_D7 : Inport  Port=6
  I_D7 : Inport  Port=7
  20l4520_MAIN : Subsystem
  Bus Creator : BusCreator  Inputs=6
  Bus Creator1 : BusCreator  Inputs=6
  Bus Creator2 : BusCreator  Inputs=7
  Bus Creator3 : BusCreator  Inputs=3
  Bus Selector : BusSelector  OutputSignals=D1_TEMP,D1_LOSS_MEAN
  Bus Selector1 : BusSelector  OutputSignals=D2_TEMP,D2_LOSS_MEAN
  Bus Selector2 : BusSelector  OutputSignals=D5_TEMP,D5_LOSS_MEAN
  Bus Selector3 : BusSelector  OutputSignals=D7_TEMP,D7_LOSS_MEAN
  Constant{,1,3,5} (4 alike) : Constant
  Constant{2,4,6..7} (4 alike) : Constant  Value=0
  Logical Operator : Logic  Operator=OR  Inputs=4  AllPortsSameDT=off  OutDataTypeStr=boolean
  Switch{,1..3} (4 alike) : Switch  Criteria=u2 > Threshold  Threshold=DIODE_204520.Junc_temp_lim  SaturateOnIntegerOverflow=off  InputSameDT=off
  D1_BUS : Outport
  D2_BUS : Outport  Port=2
  D5_BUS : Outport  Port=3
  D7_BUS : Outport  Port=4
  <D1_TEMP> : Outport  Port=5
  <D2_TEMP> : Outport  Port=6
  <D5_TEMP> : Outport  Port=7
  <D7_TEMP> : Outport  Port=8
  <D1_LOSS_MEAN> : Outport  Port=9
  <D2_LOSS_MEAN> : Outport  Port=10
  <D5_LOSS_MEAN> : Outport  Port=11
  <D7_LOSS_MEAN> : Outport  Port=12
  TEMLIM_BOOL_D : Outport  Port=13
  wires:
  20l4520_MAIN/3(D1_AVG_MEAN) -> Bus Creator/3
  20l4520_MAIN/2(D1_LOSS_MEAN) -> Bus Creator/2
  20l4520_MAIN/4(D1_AVG) -> Bus Creator/4
  20l4520_MAIN/14(D5_LOSS_MEAN) -> Bus Creator2/2
  PWM3/1 -> 20l4520_MAIN/4(PWM3)
  20l4520_MAIN/10(D2_AVG) -> Bus Creator1/4
  U_D7/1 -> 20l4520_MAIN/6(U_D7)
  20l4520_MAIN/9(D2_AVG_MEAN) -> Bus Creator1/3
  20l4520_MAIN/8(D2_LOSS_MEAN) -> Bus Creator1/2
  Bus Selector/2 -> <D1_LOSS_MEAN>/1  "<D1_LOSS_MEAN>"
  I_D7/1 -> 20l4520_MAIN/7(I_D7)
  20l4520_MAIN/18(D5_SW_MEAN) -> Bus Creator2/6
  [D2] -> Bus Selector1/1
  Switch/1 -> Logical Operator/1
  20l4520_MAIN/15(D5_LOSS) -> Bus Creator2/3
  20l4520_MAIN/13(D5_TEMP) -> Bus Creator2/1
  Bus Selector1/2 -> <D2_LOSS_MEAN>/1  "<D2_LOSS_MEAN>"
  Constant6/1 -> Switch1/3
  Logical Operator/1 -> TEMLIM_BOOL_D/1
  Bus Selector/1 -> Switch/2, <D1_TEMP>/1  "<D1_TEMP>"
  20l4520_MAIN/19(D5_SW) -> Bus Creator2/7
  Constant5/1 -> Switch1/1
  Constant7/1 -> Switch3/3
  Constant3/1 -> Switch3/1
  [D1] -> Bus Selector/1
  PWM2/1 -> 20l4520_MAIN/3(PWM2)
  20l4520_MAIN/1(D1_TEMP) -> Bus Creator/1
  20l4520_MAIN/17(D5_AVG) -> Bus Creator2/5
  20l4520_MAIN/20(D7_TEMP) -> Bus Creator3/1
  Bus Selector3/2 -> <D7_LOSS_MEAN>/1  "<D7_LOSS_MEAN>"
  [D5] -> Bus Selector2/1
  20l4520_MAIN/7(D2_TEMP) -> Bus Creator1/1
  Bus Creator3/1 -> [D7], D7_BUS/1  "D7_BUS"
  Switch2/1 -> Logical Operator/3
  20l4520_MAIN/21(D7_LOSS_MEAN) -> Bus Creator3/2
  20l4520_MAIN/16(D5_AVG_MEAN) -> Bus Creator2/4
  Bus Creator/1 -> [D1], D1_BUS/1  "D1_BUS"
  Constant4/1 -> Switch/3
  PWM4/1 -> 20l4520_MAIN/5(PWM4)
  Constant2/1 -> Switch2/3
  Bus Selector2/1 -> Switch2/2, <D5_TEMP>/1  "<D5_TEMP>"
  Switch1/1 -> Logical Operator/2
  Bus Selector1/1 -> Switch1/2, <D2_TEMP>/1  "<D2_TEMP>"
  i/1 -> 20l4520_MAIN/1(i)
  Bus Selector3/1 -> Switch3/2, <D7_TEMP>/1  "<D7_TEMP>"
  Bus Creator2/1 -> [D5], D5_BUS/1  "D5_BUS"
  20l4520_MAIN/6(D1_SW) -> Bus Creator/6
  20l4520_MAIN/5(D1_SW_MEAN) -> Bus Creator/5
  20l4520_MAIN/12(D2_SW) -> Bus Creator1/6
  Constant1/1 -> Switch2/1
  Switch3/1 -> Logical Operator/4
  20l4520_MAIN/22(D7_LOSS) -> Bus Creator3/3
  [D7] -> Bus Selector3/1
  PWM1/1 -> 20l4520_MAIN/2(PWM1)
  Bus Creator1/1 -> [D2], D2_BUS/1  "D2_BUS"
  20l4520_MAIN/11(D2_SW_MEAN) -> Bus Creator1/5
  Constant/1 -> Switch/1
  Bus Selector2/2 -> <D5_LOSS_MEAN>/1  "<D5_LOSS_MEAN>"

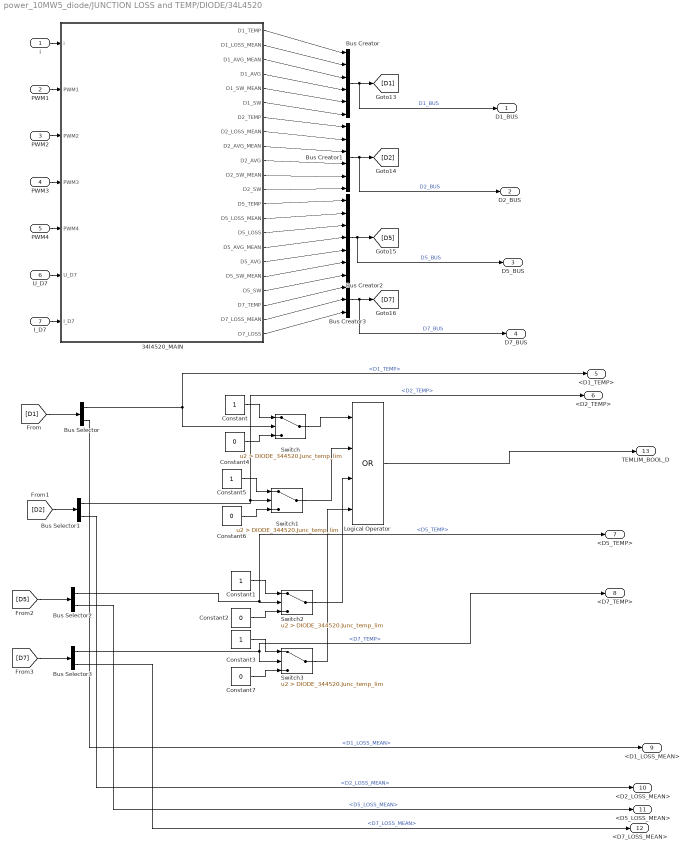
== system power_10MW5_diode/JUNCTION LOSS and TEMP/DIODE/34L4520 ==
  i : Inport
  PWM1 : Inport  Port=2
  PWM2 : Inport  Port=3
  PWM3 : Inport  Port=4
  PWM4 : Inport  Port=5
  U_D7 : Inport  Port=6
  I_D7 : Inport  Port=7
  34l4520_MAIN : Subsystem
  Bus Creator : BusCreator  Inputs=6
  Bus Creator1 : BusCreator  Inputs=6
  Bus Creator2 : BusCreator  Inputs=7
  Bus Creator3 : BusCreator  Inputs=3
  Bus Selector : BusSelector  OutputSignals=D1_TEMP,D1_LOSS_MEAN
  Bus Selector1 : BusSelector  OutputSignals=D2_TEMP,D2_LOSS_MEAN
  Bus Selector2 : BusSelector  OutputSignals=D5_TEMP,D5_LOSS_MEAN
  Bus Selector3 : BusSelector  OutputSignals=D7_TEMP,D7_LOSS_MEAN
  Constant{,1,3,5} (4 alike) : Constant
  Constant{2,4,6..7} (4 alike) : Constant  Value=0
  Logical Operator : Logic  Operator=OR  Inputs=4  AllPortsSameDT=off  OutDataTypeStr=boolean
  Switch{,1..3} (4 alike) : Switch  Criteria=u2 > Threshold  Threshold=DIODE_344520.Junc_temp_lim  SaturateOnIntegerOverflow=off  InputSameDT=off
  D1_BUS : Outport
  D2_BUS : Outport  Port=2
  D5_BUS : Outport  Port=3
  D7_BUS : Outport  Port=4
  <D1_TEMP> : Outport  Port=5
  <D2_TEMP> : Outport  Port=6
  <D5_TEMP> : Outport  Port=7
  <D7_TEMP> : Outport  Port=8
  <D1_LOSS_MEAN> : Outport  Port=9
  <D2_LOSS_MEAN> : Outport  Port=10
  <D5_LOSS_MEAN> : Outport  Port=11
  <D7_LOSS_MEAN> : Outport  Port=12
  TEMLIM_BOOL_D : Outport  Port=13
  wires:
  Bus Selector2/2 -> <D5_LOSS_MEAN>/1  "<D5_LOSS_MEAN>"
  Constant/1 -> Switch/1
  34l4520_MAIN/11(D2_SW_MEAN) -> Bus Creator1/5
  Bus Creator1/1 -> D2_BUS/1, [D2]  "D2_BUS"
  PWM1/1 -> 34l4520_MAIN/2(PWM1)
  [D7] -> Bus Selector3/1
  34l4520_MAIN/22(D7_LOSS) -> Bus Creator3/3
  Switch3/1 -> Logical Operator/4
  Constant1/1 -> Switch2/1
  34l4520_MAIN/12(D2_SW) -> Bus Creator1/6
  34l4520_MAIN/5(D1_SW_MEAN) -> Bus Creator/5
  34l4520_MAIN/6(D1_SW) -> Bus Creator/6
  Bus Creator2/1 -> D5_BUS/1, [D5]  "D5_BUS"
  Bus Selector3/1 -> <D7_TEMP>/1, Switch3/2  "<D7_TEMP>"
  i/1 -> 34l4520_MAIN/1(i)
  Bus Selector1/1 -> <D2_TEMP>/1, Switch1/2  "<D2_TEMP>"
  Switch1/1 -> Logical Operator/2
  Bus Selector2/1 -> <D5_TEMP>/1, Switch2/2  "<D5_TEMP>"
  Constant2/1 -> Switch2/3
  PWM4/1 -> 34l4520_MAIN/5(PWM4)
  Constant4/1 -> Switch/3
  Bus Creator/1 -> D1_BUS/1, [D1]  "D1_BUS"
  34l4520_MAIN/16(D5_AVG_MEAN) -> Bus Creator2/4
  34l4520_MAIN/21(D7_LOSS_MEAN) -> Bus Creator3/2
  Switch2/1 -> Logical Operator/3
  Bus Creator3/1 -> D7_BUS/1, [D7]  "D7_BUS"
  34l4520_MAIN/7(D2_TEMP) -> Bus Creator1/1
  [D5] -> Bus Selector2/1
  Bus Selector3/2 -> <D7_LOSS_MEAN>/1  "<D7_LOSS_MEAN>"
  34l4520_MAIN/20(D7_TEMP) -> Bus Creator3/1
  34l4520_MAIN/17(D5_AVG) -> Bus Creator2/5
  34l4520_MAIN/1(D1_TEMP) -> Bus Creator/1
  PWM2/1 -> 34l4520_MAIN/3(PWM2)
  [D1] -> Bus Selector/1
  Constant3/1 -> Switch3/1
  Constant7/1 -> Switch3/3
  Constant5/1 -> Switch1/1
  34l4520_MAIN/19(D5_SW) -> Bus Creator2/7
  Bus Selector/1 -> <D1_TEMP>/1, Switch/2  "<D1_TEMP>"
  Logical Operator/1 -> TEMLIM_BOOL_D/1
  Constant6/1 -> Switch1/3
  Bus Selector1/2 -> <D2_LOSS_MEAN>/1  "<D2_LOSS_MEAN>"
  34l4520_MAIN/13(D5_TEMP) -> Bus Creator2/1
  34l4520_MAIN/15(D5_LOSS) -> Bus Creator2/3
  Switch/1 -> Logical Operator/1
  [D2] -> Bus Selector1/1
  34l4520_MAIN/18(D5_SW_MEAN) -> Bus Creator2/6
  I_D7/1 -> 34l4520_MAIN/7(I_D7)
  Bus Selector/2 -> <D1_LOSS_MEAN>/1  "<D1_LOSS_MEAN>"
  34l4520_MAIN/8(D2_LOSS_MEAN) -> Bus Creator1/2
  34l4520_MAIN/9(D2_AVG_MEAN) -> Bus Creator1/3
  U_D7/1 -> 34l4520_MAIN/6(U_D7)
  34l4520_MAIN/10(D2_AVG) -> Bus Creator1/4
  PWM3/1 -> 34l4520_MAIN/4(PWM3)
  34l4520_MAIN/14(D5_LOSS_MEAN) -> Bus Creator2/2
  34l4520_MAIN/4(D1_AVG) -> Bus Creator/4
  34l4520_MAIN/2(D1_LOSS_MEAN) -> Bus Creator/2
  34l4520_MAIN/3(D1_AVG_MEAN) -> Bus Creator/3

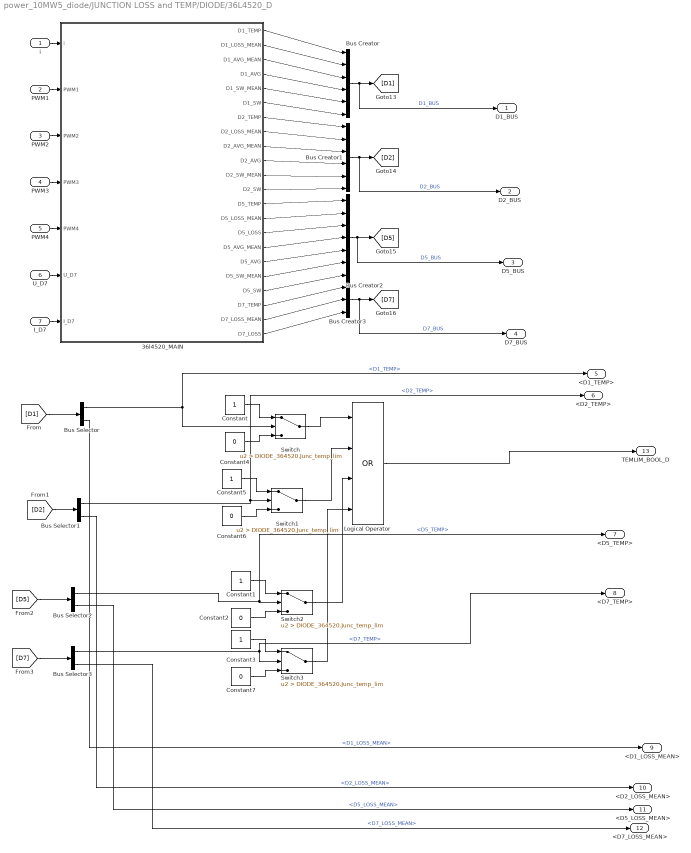
== system power_10MW5_diode/JUNCTION LOSS and TEMP/DIODE/36L4520_D ==
  i : Inport
  PWM1 : Inport  Port=2
  PWM2 : Inport  Port=3
  PWM3 : Inport  Port=4
  PWM4 : Inport  Port=5
  U_D7 : Inport  Port=6
  I_D7 : Inport  Port=7
  36l4520_MAIN : Subsystem
  Bus Creator : BusCreator  Inputs=6
  Bus Creator1 : BusCreator  Inputs=6
  Bus Creator2 : BusCreator  Inputs=7
  Bus Creator3 : BusCreator  Inputs=3
  Bus Selector : BusSelector  OutputSignals=D1_TEMP,D1_LOSS_MEAN
  Bus Selector1 : BusSelector  OutputSignals=D2_TEMP,D2_LOSS_MEAN
  Bus Selector2 : BusSelector  OutputSignals=D5_TEMP,D5_LOSS_MEAN
  Bus Selector3 : BusSelector  OutputSignals=D7_TEMP,D7_LOSS_MEAN
  Constant{,1,3,5} (4 alike) : Constant
  Constant{2,4,6..7} (4 alike) : Constant  Value=0
  Logical Operator : Logic  Operator=OR  Inputs=4  AllPortsSameDT=off  OutDataTypeStr=boolean
  Switch{,1..3} (4 alike) : Switch  Criteria=u2 > Threshold  Threshold=DIODE_364520.Junc_temp_lim  SaturateOnIntegerOverflow=off  InputSameDT=off
  D1_BUS : Outport
  D2_BUS : Outport  Port=2
  D5_BUS : Outport  Port=3
  D7_BUS : Outport  Port=4
  <D1_TEMP> : Outport  Port=5
  <D2_TEMP> : Outport  Port=6
  <D5_TEMP> : Outport  Port=7
  <D7_TEMP> : Outport  Port=8
  <D1_LOSS_MEAN> : Outport  Port=9
  <D2_LOSS_MEAN> : Outport  Port=10
  <D5_LOSS_MEAN> : Outport  Port=11
  <D7_LOSS_MEAN> : Outport  Port=12
  TEMLIM_BOOL_D : Outport  Port=13
  wires:
  36l4520_MAIN/3(D1_AVG_MEAN) -> Bus Creator/3
  36l4520_MAIN/2(D1_LOSS_MEAN) -> Bus Creator/2
  36l4520_MAIN/4(D1_AVG) -> Bus Creator/4
  36l4520_MAIN/14(D5_LOSS_MEAN) -> Bus Creator2/2
  PWM3/1 -> 36l4520_MAIN/4(PWM3)
  36l4520_MAIN/10(D2_AVG) -> Bus Creator1/4
  U_D7/1 -> 36l4520_MAIN/6(U_D7)
  36l4520_MAIN/9(D2_AVG_MEAN) -> Bus Creator1/3
  36l4520_MAIN/8(D2_LOSS_MEAN) -> Bus Creator1/2
  Bus Selector/2 -> <D1_LOSS_MEAN>/1  "<D1_LOSS_MEAN>"
  I_D7/1 -> 36l4520_MAIN/7(I_D7)
  36l4520_MAIN/18(D5_SW_MEAN) -> Bus Creator2/6
  [D2] -> Bus Selector1/1
  Switch/1 -> Logical Operator/1
  36l4520_MAIN/15(D5_LOSS) -> Bus Creator2/3
  36l4520_MAIN/13(D5_TEMP) -> Bus Creator2/1
  Bus Selector1/2 -> <D2_LOSS_MEAN>/1  "<D2_LOSS_MEAN>"
  Constant6/1 -> Switch1/3
  Logical Operator/1 -> TEMLIM_BOOL_D/1
  Bus Selector/1 -> Switch/2, <D1_TEMP>/1  "<D1_TEMP>"
  36l4520_MAIN/19(D5_SW) -> Bus Creator2/7
  Constant5/1 -> Switch1/1
  Constant7/1 -> Switch3/3
  Constant3/1 -> Switch3/1
  [D1] -> Bus Selector/1
  PWM2/1 -> 36l4520_MAIN/3(PWM2)
  36l4520_MAIN/1(D1_TEMP) -> Bus Creator/1
  36l4520_MAIN/17(D5_AVG) -> Bus Creator2/5
  36l4520_MAIN/20(D7_TEMP) -> Bus Creator3/1
  Bus Selector3/2 -> <D7_LOSS_MEAN>/1  "<D7_LOSS_MEAN>"
  [D5] -> Bus Selector2/1
  36l4520_MAIN/7(D2_TEMP) -> Bus Creator1/1
  Bus Creator3/1 -> [D7], D7_BUS/1  "D7_BUS"
  Switch2/1 -> Logical Operator/3
  36l4520_MAIN/21(D7_LOSS_MEAN) -> Bus Creator3/2
  36l4520_MAIN/16(D5_AVG_MEAN) -> Bus Creator2/4
  Bus Creator/1 -> [D1], D1_BUS/1  "D1_BUS"
  Constant4/1 -> Switch/3
  PWM4/1 -> 36l4520_MAIN/5(PWM4)
  Constant2/1 -> Switch2/3
  Bus Selector2/1 -> Switch2/2, <D5_TEMP>/1  "<D5_TEMP>"
  Switch1/1 -> Logical Operator/2
  Bus Selector1/1 -> Switch1/2, <D2_TEMP>/1  "<D2_TEMP>"
  i/1 -> 36l4520_MAIN/1(i)
  Bus Selector3/1 -> Switch3/2, <D7_TEMP>/1  "<D7_TEMP>"
  Bus Creator2/1 -> [D5], D5_BUS/1  "D5_BUS"
  36l4520_MAIN/6(D1_SW) -> Bus Creator/6
  36l4520_MAIN/5(D1_SW_MEAN) -> Bus Creator/5
  36l4520_MAIN/12(D2_SW) -> Bus Creator1/6
  Constant1/1 -> Switch2/1
  Switch3/1 -> Logical Operator/4
  36l4520_MAIN/22(D7_LOSS) -> Bus Creator3/3
  [D7] -> Bus Selector3/1
  PWM1/1 -> 36l4520_MAIN/2(PWM1)
  Bus Creator1/1 -> [D2], D2_BUS/1  "D2_BUS"
  36l4520_MAIN/11(D2_SW_MEAN) -> Bus Creator1/5
  Constant/1 -> Switch/1
  Bus Selector2/2 -> <D5_LOSS_MEAN>/1  "<D5_LOSS_MEAN>"
